simulink model "eVTOL_System"  (R2024b)
settings: Solver=FixedStepAuto  StartTime=0.0  StopTime=inf  RelTol=1e-3
undefined symbols (not defined in the file): airspeed, Battery, BCE12, BCE_Set_init, BMS_Controller_State, C, Cell10_P, Cell11_P, Cell12_P, Cell13_P, Cell14_P, Cell15_P, Cell16_P, Cell17_P, Cell18_P, Cell19_P, Cell1_N, Cell1_P, Cell20_P, Cell21_P, Cell22_P, Cell23_P, Cell24_P, Cell2_P, Cell3_P, Cell4_P, Cell5_P, Cell6_P, Cell7_P, Cell8_P, Cell9_P, Charging_State, CityMission, control, controlParams, ControlSampleTime, CriticalTiltAngle, currentFactor, CV_Gain, ddx, ddy, ddz, Device_01, Device_02, DiscIntNeverNeededParam, dx, dy, dz, Earth, env, F, F28379D_ADC_MaxCount, F28379D_ADC_Vmax, FixedWingMission, flightState, Foc_Ki_IxTcpu, Foc_Ki_S, Foc_Kp_I, Foc_Kp_S, fractalcoef ... (+68)
libraries: fl_lib x1115, nesl_utility x617, slrealtimeethercatlib x217, simulink x130, canmsglib x101, speedgoatlib_IO611_obsolete x91, slpidlib x49, mcbcontrolslib x44, slrealtimeutilitieslib x35, speedgoatlib_hdlCoder_IO3xx x31, dspstat3 x24, mcbpositiondecoderlib x12
(part 21 of 31)

== system eVTOL_System/Flight Controller/Autopilot/Fixed Wing Controller/Fixed Wing Controller Tuning/Attitude Controller/Pitch Roll Controller ==
  note: Small angle assumption. x axis body rate = rate of roll
  note: Inspired by PX4's fixed wing controller
      | https://docs.px4.io/master/en/flight_stack/controller_diagrams.html
  Pitch SP : Inport
  Roll SP : Inport  Port=2
  YPR : Inport  Port=3
  Ang Rate : Inport  Port=4
  Airspeed : Inport  Port=5
  Enable : EnablePort
  Demux : Demux  Outputs=3
  Demux1 : Demux  Outputs=3
  Mux : Mux  Inputs=3
  Pitch Angle Controller : slpidlib/PID Controller  Controller=PID  Form=Parallel  TimeDomain=Discrete-time  UseExternalTs=off  SampleTime=0.005  IntegratorMethod=Forward Euler  FilterMethod=Forward Euler  ControllerParametersSource=internal  P=17.6399272009125  I=10.1914925604101  UseKiTs=off  D=1.4272793655692  UseExternalDerivativeSource=off  N=0.16530941788163  UseFilter=on  TunerSelectOption=Transfer Function Based (PID Tuner App)  InitialConditionSource=internal  InitialConditionForIntegrator=0  InitialConditionForFilter=0  DifferentiatorICPrevScaledInput=0  ExternalReset=none  TrackingMode=off  Kt=1  LimitOutput=on  SatLimitsSource=internal  UpperSaturationLimit=inf  LowerSaturationLimit=-inf  LinearizeAsGain=on  AntiWindupMode=clamping  Kb=1  LimitIntegrator=off  UpperIntegratorSaturationLimit=inf  LowerIntegratorSaturationLimit=-inf  POutMin=[]  POutMax=[]  IOutMin=[]  IOutMax=[]  DOutMin=[]  DOutMax=[]  NOutMin=[]  NOutMax=[]  SumOutMin=[]  SumOutMax=[]  SaturationOutMin=[]  SaturationOutMax=[]  PParamMin=[]  PParamMax=[]  IParamMin=[]  IParamMax=[]  DParamMin=[]  DParamMax=[]  NParamMin=[]  NParamMax=[]  KbParamMin=[]  KbParamMax=[]  KtParamMin=[]  KtParamMax=[]  KbOutMin=[]  KbOutMax=[]  KtOutMin=[]  KtOutMax=[]  IntegratorOutMin=[]  IntegratorOutMax=[]  FilterOutMin=[]  FilterOutMax=[]  SumI1OutMin=[]  SumI1OutMax=[]  SumI2OutMin=[]  SumI2OutMax=[]  SumI3OutMin=[]  SumI3OutMax=[]  SumI4OutMin=[]  SumI4OutMax=[]  SumDOutMin=[]  SumDOutMax=[]  DifferentiatorOutMin=[]  DifferentiatorOutMax=[]  FilterDiffOutCoefMin=[]  FilterDiffOutCoefMax=[]  ReciprocalOutMin=[]  ReciprocalOutMax=[]  SumDenOutMin=[]  SumDenOutMax=[]  SumNumOutMin=[]  SumNumOutMax=[]  DivideOutMin=[]  DivideOutMax=[]  UdiffTsProdOutMin=[]  UdiffTsProdOutMax=[]  NTsProdOutMin=[]  NTsProdOutMax=[]  UintegralTsProdOutMin=[]  UintegralTsProdOutMax=[]  UngainTsProdOutMin=[]  UngainTsProdOutMax=[]  ClampingZeroOutDataTypeStr=Inherit: Inherit via back propagation  ClampingZeroOutMin=[]  ClampingZeroOutMax=[]  FilterDenConstantOutDataTypeStr=Inherit: Inherit via back propagation  FilterDenConstantOutMin=[]  FilterDenConstantOutMax=[]  PCopyOutDataTypeStr=Inherit: Inherit via back propagation  PCopyOutMin=[]  PCopyOutMax=[]  NCopyOutDataTypeStr=Inherit: Inherit via back propagation  NCopyOutMin=[]  NCopyOutMax=[]  IntegratorContinuousStateAttributes=''  IntegratorStateMustResolveToSignalObject=off  IntegratorRTWStateStorageClass=Auto  FilterContinuousStateAttributes=''  FilterStateMustResolveToSignalObject=off  FilterRTWStateStorageClass=Auto  ParallelPVariant=InternalParameters  IdealPVariant=Disabled  IVariant=InternalParameters  DVariant=InternalParameters  IntegratorVariant=Discrete  SatVariant=Enabled  AWVariant=DiscClampingParallel  PCopyVariant=Disabled  TRVariant=Disabled  FdbkBlocksVariant=Forward  IdealPFdbkVariant=Disabled  SatFdbkVariant=Disabled  DerivativeFilterVariant=ForwardEulerFilter  NVariant=InternalParameters  NCopyVariant=Disabled  FilterICVariant=InternalICsFilter  IntegratorICVariant=InternalICs  ExternalResetVariant=Disabled  TRSumVariant=Passthrough  SumFdbkVariant=Disabled  SumVariant=Sum_PID  TsampFilterVariant=InternalTs  TsampNgainVariant=Passthrough  TsampIntegralVariant=Disabled_SignalSpec  ExternalSaturationOutDataTypeStr=Inherit: Same as second input  DerivativeSourceVariant=ErrorSignal  PreIntVariant=InternalPreInt
  Pitch Rate Controller : slpidlib/PID Controller  Controller=P  Form=Parallel  TimeDomain=Discrete-time  UseExternalTs=off  SampleTime=0.005  IntegratorMethod=Forward Euler  FilterMethod=Forward Euler  ControllerParametersSource=internal  P=0.198532533167891  I=0  UseKiTs=off  D=0  UseExternalDerivativeSource=off  N=100  UseFilter=on  TunerSelectOption=Transfer Function Based (PID Tuner App)  InitialConditionSource=internal  InitialConditionForIntegrator=0  InitialConditionForFilter=0  DifferentiatorICPrevScaledInput=0  ExternalReset=either  TrackingMode=off  Kt=1  LimitOutput=on  SatLimitsSource=internal  UpperSaturationLimit=inf  LowerSaturationLimit=-inf  LinearizeAsGain=on  AntiWindupMode=clamping  Kb=1  LimitIntegrator=off  UpperIntegratorSaturationLimit=inf  LowerIntegratorSaturationLimit=-inf  POutMin=[]  POutMax=[]  IOutMin=[]  IOutMax=[]  DOutMin=[]  DOutMax=[]  NOutMin=[]  NOutMax=[]  SumOutMin=[]  SumOutMax=[]  SaturationOutMin=[]  SaturationOutMax=[]  PParamMin=[]  PParamMax=[]  IParamMin=[]  IParamMax=[]  DParamMin=[]  DParamMax=[]  NParamMin=[]  NParamMax=[]  KbParamMin=[]  KbParamMax=[]  KtParamMin=[]  KtParamMax=[]  KbOutMin=[]  KbOutMax=[]  KtOutMin=[]  KtOutMax=[]  IntegratorOutMin=[]  IntegratorOutMax=[]  FilterOutMin=[]  FilterOutMax=[]  SumI1OutMin=[]  SumI1OutMax=[]  SumI2OutMin=[]  SumI2OutMax=[]  SumI3OutMin=[]  SumI3OutMax=[]  SumI4OutMin=[]  SumI4OutMax=[]  SumDOutMin=[]  SumDOutMax=[]  DifferentiatorOutMin=[]  DifferentiatorOutMax=[]  FilterDiffOutCoefMin=[]  FilterDiffOutCoefMax=[]  ReciprocalOutMin=[]  ReciprocalOutMax=[]  SumDenOutMin=[]  SumDenOutMax=[]  SumNumOutMin=[]  SumNumOutMax=[]  DivideOutMin=[]  DivideOutMax=[]  UdiffTsProdOutMin=[]  UdiffTsProdOutMax=[]  NTsProdOutMin=[]  NTsProdOutMax=[]  UintegralTsProdOutMin=[]  UintegralTsProdOutMax=[]  UngainTsProdOutMin=[]  UngainTsProdOutMax=[]  ClampingZeroOutDataTypeStr=Inherit: Inherit via back propagation  ClampingZeroOutMin=[]  ClampingZeroOutMax=[]  FilterDenConstantOutDataTypeStr=Inherit: Inherit via back propagation  FilterDenConstantOutMin=[]  FilterDenConstantOutMax=[]  PCopyOutDataTypeStr=Inherit: Inherit via back propagation  PCopyOutMin=[]  PCopyOutMax=[]  NCopyOutDataTypeStr=Inherit: Inherit via back propagation  NCopyOutMin=[]  NCopyOutMax=[]  IntegratorContinuousStateAttributes=''  IntegratorStateMustResolveToSignalObject=off  IntegratorRTWStateStorageClass=Auto  FilterContinuousStateAttributes=''  FilterStateMustResolveToSignalObject=off  FilterRTWStateStorageClass=Auto  ParallelPVariant=InternalParameters  IdealPVariant=Disabled  IVariant=Disabled  DVariant=Disabled  IntegratorVariant=Disabled  SatVariant=Enabled  AWVariant=Disabled  PCopyVariant=Disabled  TRVariant=Disabled  FdbkBlocksVariant=Forward  IdealPFdbkVariant=Disabled  SatFdbkVariant=Disabled  DerivativeFilterVariant=Disabled  NVariant=Disabled  NCopyVariant=Disabled_SignalSpec  FilterICVariant=Disabled  IntegratorICVariant=Disabled  ExternalResetVariant=Disabled  TRSumVariant=Passthrough  SumFdbkVariant=Disabled  SumVariant=Passthrough_P  TsampFilterVariant=InternalTs  TsampNgainVariant=Passthrough  TsampIntegralVariant=Disabled_SignalSpec  ExternalSaturationOutDataTypeStr=Inherit: Same as second input  DerivativeSourceVariant=Disabled  PreIntVariant=InternalPreInt
  Roll Angle Controller : slpidlib/PID Controller  Controller=P  Form=Parallel  TimeDomain=Discrete-time  UseExternalTs=off  SampleTime=0.005  IntegratorMethod=Forward Euler  FilterMethod=Forward Euler  ControllerParametersSource=internal  P=10.1019363886622  I=0.5  UseKiTs=off  D=2  UseExternalDerivativeSource=off  N=100  UseFilter=on  TunerSelectOption=Transfer Function Based (PID Tuner App)  InitialConditionSource=internal  InitialConditionForIntegrator=0  InitialConditionForFilter=0  DifferentiatorICPrevScaledInput=0  ExternalReset=none  TrackingMode=off  Kt=1  LimitOutput=on  SatLimitsSource=internal  UpperSaturationLimit=control.maxRollRate  LowerSaturationLimit=control.minRollRate  LinearizeAsGain=on  AntiWindupMode=clamping  Kb=1  LimitIntegrator=off  UpperIntegratorSaturationLimit=inf  LowerIntegratorSaturationLimit=-inf  POutMin=[]  POutMax=[]  IOutMin=[]  IOutMax=[]  DOutMin=[]  DOutMax=[]  NOutMin=[]  NOutMax=[]  SumOutMin=[]  SumOutMax=[]  SaturationOutMin=[]  SaturationOutMax=[]  PParamMin=[]  PParamMax=[]  IParamMin=[]  IParamMax=[]  DParamMin=[]  DParamMax=[]  NParamMin=[]  NParamMax=[]  KbParamMin=[]  KbParamMax=[]  KtParamMin=[]  KtParamMax=[]  KbOutMin=[]  KbOutMax=[]  KtOutMin=[]  KtOutMax=[]  IntegratorOutMin=[]  IntegratorOutMax=[]  FilterOutMin=[]  FilterOutMax=[]  SumI1OutMin=[]  SumI1OutMax=[]  SumI2OutMin=[]  SumI2OutMax=[]  SumI3OutMin=[]  SumI3OutMax=[]  SumI4OutMin=[]  SumI4OutMax=[]  SumDOutMin=[]  SumDOutMax=[]  DifferentiatorOutMin=[]  DifferentiatorOutMax=[]  FilterDiffOutCoefMin=[]  FilterDiffOutCoefMax=[]  ReciprocalOutMin=[]  ReciprocalOutMax=[]  SumDenOutMin=[]  SumDenOutMax=[]  SumNumOutMin=[]  SumNumOutMax=[]  DivideOutMin=[]  DivideOutMax=[]  UdiffTsProdOutMin=[]  UdiffTsProdOutMax=[]  NTsProdOutMin=[]  NTsProdOutMax=[]  UintegralTsProdOutMin=[]  UintegralTsProdOutMax=[]  UngainTsProdOutMin=[]  UngainTsProdOutMax=[]  ClampingZeroOutDataTypeStr=Inherit: Inherit via back propagation  ClampingZeroOutMin=[]  ClampingZeroOutMax=[]  FilterDenConstantOutDataTypeStr=Inherit: Inherit via back propagation  FilterDenConstantOutMin=[]  FilterDenConstantOutMax=[]  PCopyOutDataTypeStr=Inherit: Inherit via back propagation  PCopyOutMin=[]  PCopyOutMax=[]  NCopyOutDataTypeStr=Inherit: Inherit via back propagation  NCopyOutMin=[]  NCopyOutMax=[]  IntegratorContinuousStateAttributes=''  IntegratorStateMustResolveToSignalObject=off  IntegratorRTWStateStorageClass=Auto  FilterContinuousStateAttributes=''  FilterStateMustResolveToSignalObject=off  FilterRTWStateStorageClass=Auto  ParallelPVariant=InternalParameters  IdealPVariant=Disabled  IVariant=Disabled  DVariant=Disabled  IntegratorVariant=Disabled  SatVariant=Enabled  AWVariant=Disabled  PCopyVariant=Disabled  TRVariant=Disabled  FdbkBlocksVariant=Forward  IdealPFdbkVariant=Disabled  SatFdbkVariant=Disabled  DerivativeFilterVariant=Disabled  NVariant=Disabled  NCopyVariant=Disabled_SignalSpec  FilterICVariant=Disabled  IntegratorICVariant=Disabled  ExternalResetVariant=Disabled  TRSumVariant=Passthrough  SumFdbkVariant=Disabled  SumVariant=Passthrough_P  TsampFilterVariant=InternalTs  TsampNgainVariant=Passthrough  TsampIntegralVariant=Disabled_SignalSpec  ExternalSaturationOutDataTypeStr=Inherit: Same as second input  DerivativeSourceVariant=Disabled  PreIntVariant=InternalPreInt
  Roll Rate Controller : slpidlib/PID Controller  Controller=PI  Form=Parallel  TimeDomain=Discrete-time  UseExternalTs=off  SampleTime=0.005  IntegratorMethod=Forward Euler  FilterMethod=Forward Euler  ControllerParametersSource=internal  P=0.1457375768301  I=3.00000582031009  UseKiTs=off  D=2  UseExternalDerivativeSource=off  N=100  UseFilter=on  TunerSelectOption=Transfer Function Based (PID Tuner App)  InitialConditionSource=internal  InitialConditionForIntegrator=0  InitialConditionForFilter=0  DifferentiatorICPrevScaledInput=0  ExternalReset=none  TrackingMode=off  Kt=1  LimitOutput=on  SatLimitsSource=internal  UpperSaturationLimit=1  LowerSaturationLimit=-1  LinearizeAsGain=on  AntiWindupMode=clamping  Kb=1  LimitIntegrator=off  UpperIntegratorSaturationLimit=inf  LowerIntegratorSaturationLimit=-inf  POutMin=[]  POutMax=[]  IOutMin=[]  IOutMax=[]  DOutMin=[]  DOutMax=[]  NOutMin=[]  NOutMax=[]  SumOutMin=[]  SumOutMax=[]  SaturationOutMin=[]  SaturationOutMax=[]  PParamMin=[]  PParamMax=[]  IParamMin=[]  IParamMax=[]  DParamMin=[]  DParamMax=[]  NParamMin=[]  NParamMax=[]  KbParamMin=[]  KbParamMax=[]  KtParamMin=[]  KtParamMax=[]  KbOutMin=[]  KbOutMax=[]  KtOutMin=[]  KtOutMax=[]  IntegratorOutMin=[]  IntegratorOutMax=[]  FilterOutMin=[]  FilterOutMax=[]  SumI1OutMin=[]  SumI1OutMax=[]  SumI2OutMin=[]  SumI2OutMax=[]  SumI3OutMin=[]  SumI3OutMax=[]  SumI4OutMin=[]  SumI4OutMax=[]  SumDOutMin=[]  SumDOutMax=[]  DifferentiatorOutMin=[]  DifferentiatorOutMax=[]  FilterDiffOutCoefMin=[]  FilterDiffOutCoefMax=[]  ReciprocalOutMin=[]  ReciprocalOutMax=[]  SumDenOutMin=[]  SumDenOutMax=[]  SumNumOutMin=[]  SumNumOutMax=[]  DivideOutMin=[]  DivideOutMax=[]  UdiffTsProdOutMin=[]  UdiffTsProdOutMax=[]  NTsProdOutMin=[]  NTsProdOutMax=[]  UintegralTsProdOutMin=[]  UintegralTsProdOutMax=[]  UngainTsProdOutMin=[]  UngainTsProdOutMax=[]  ClampingZeroOutDataTypeStr=Inherit: Inherit via back propagation  ClampingZeroOutMin=[]  ClampingZeroOutMax=[]  FilterDenConstantOutDataTypeStr=Inherit: Inherit via back propagation  FilterDenConstantOutMin=[]  FilterDenConstantOutMax=[]  PCopyOutDataTypeStr=Inherit: Inherit via back propagation  PCopyOutMin=[]  PCopyOutMax=[]  NCopyOutDataTypeStr=Inherit: Inherit via back propagation  NCopyOutMin=[]  NCopyOutMax=[]  IntegratorContinuousStateAttributes=''  IntegratorStateMustResolveToSignalObject=off  IntegratorRTWStateStorageClass=Auto  FilterContinuousStateAttributes=''  FilterStateMustResolveToSignalObject=off  FilterRTWStateStorageClass=Auto  ParallelPVariant=InternalParameters  IdealPVariant=Disabled  IVariant=InternalParameters  DVariant=Disabled  IntegratorVariant=Discrete  SatVariant=Enabled  AWVariant=DiscClampingParallel  PCopyVariant=Disabled  TRVariant=Disabled  FdbkBlocksVariant=Forward  IdealPFdbkVariant=Disabled  SatFdbkVariant=Disabled  DerivativeFilterVariant=Disabled  NVariant=Disabled  NCopyVariant=Disabled_SignalSpec  FilterICVariant=Disabled  IntegratorICVariant=InternalICs  ExternalResetVariant=Disabled  TRSumVariant=Passthrough  SumFdbkVariant=Disabled  SumVariant=Sum_PI  TsampFilterVariant=InternalTs  TsampNgainVariant=Passthrough  TsampIntegralVariant=Disabled_SignalSpec  ExternalSaturationOutDataTypeStr=Inherit: Same as second input  DerivativeSourceVariant=Disabled  PreIntVariant=InternalPreInt
  Saturation : Saturate  UpperLimit=control.maxRoll  LowerLimit=control.minRoll
  Saturation1 : Saturate  UpperLimit=control.maxPitch  LowerLimit=control.minPitch
  Saturation2 : Saturate  UpperLimit=0.3  LowerLimit=-0.3
  Sum{,1..3} (4 alike) : Sum  Inputs=|+-
  Terminator : Terminator
  Turn Coordinator : Subsystem
  Unary Minus1 : UnaryMinus
  AER : Outport
  wires:
  Sum/1 -> Pitch Angle Controller/1
  YPR/1 -> Demux/1
  Demux/2 -> Sum/2
  Mux/1 -> AER/1
  Saturation1/1 -> Sum/1, Turn Coordinator/2(Pitch SP)
  Ang Rate/1 -> Demux1/1
  Pitch SP/1 -> Saturation1/1
  Pitch Rate Controller/1 -> Unary Minus1/1
  Demux/3 -> Sum1/2
  Saturation/1 -> Sum1/1, Turn Coordinator/1(Roll SP)
  Roll SP/1 -> Saturation/1
  Sum1/1 -> Roll Angle Controller/1
  Demux/1 -> Terminator/1
  Airspeed/1 -> Turn Coordinator/3(Airspeed)
  Demux1/3 -> Turn Coordinator/4(r)
  Turn Coordinator/1(Rudder) -> Mux/3  "dR"
  Unary Minus1/1 -> Mux/2  "dE"
  Saturation2/1 -> Mux/1
  Sum2/1 -> Roll Rate Controller/1
  Roll Angle Controller/1 -> Sum2/1
  Demux1/1 -> Sum2/2
  Roll Rate Controller/1 -> Saturation2/1
  Demux1/2 -> Sum3/2
  Pitch Angle Controller/1 -> Sum3/1
  Sum3/1 -> Pitch Rate Controller/1

== system eVTOL_System/Flight Controller/Autopilot/Fixed Wing Controller/Fixed Wing Controller Tuning/Attitude Controller/Rudder Heading Controller ==
  note: Rudder control during takeoff ground-run.
      | Not implemented currently.
  Yaw SP : Inport
  YPR : Inport  Port=2
  Ang Rate : Inport  Port=3
  Enable : EnablePort
  Constant : Constant  Value=0
  Constant1 : Constant  Value=0
  Mux : Mux  Inputs=3
  Selector : Selector  InputPortWidth=3  IndexOptions=Index vector (dialog)  Indices=1  OutputSizes=1
  Selector1 : Selector  InputPortWidth=3  IndexOptions=Index vector (dialog)  Indices=3  OutputSizes=1
  Terminator : Terminator
  Terminator1 : Terminator
  Terminator2 : Terminator
  AER : Outport
  wires:
  YPR/1 -> Selector/1
  Mux/1 -> AER/1
  Constant/1 -> Mux/2, Mux/1
  Ang Rate/1 -> Selector1/1
  Constant1/1 -> Mux/3
  Yaw SP/1 -> Terminator/1
  Selector/1 -> Terminator1/1
  Selector1/1 -> Terminator2/1

== system eVTOL_System/Flight Controller/Autopilot/Multicopter Controller/Attitude Control/Derivative Gain/Pitch Ref Deriv ==
  In1 : Inport
  Discrete-Time Integrator : DiscreteIntegrator  SampleTime=-1  ICPrevOutput=DiscIntNeverNeededParam  ICPrevScaledInput=DiscIntNeverNeededParam
  Gain : Gain  Gain=controlParams.N_PITCH
  Sum : Sum  Inputs=|+-
  Out1 : Outport
  wires:
  Gain/1 -> Out1/1, Discrete-Time Integrator/1
  In1/1 -> Sum/1
  Sum/1 -> Gain/1
  Discrete-Time Integrator/1 -> Sum/2

== system eVTOL_System/Flight Controller/Autopilot/Multicopter Controller/Attitude Control/Derivative Gain/Roll Ref Deriv ==
  In1 : Inport
  Discrete-Time Integrator : DiscreteIntegrator  SampleTime=-1  ICPrevOutput=DiscIntNeverNeededParam  ICPrevScaledInput=DiscIntNeverNeededParam
  Gain : Gain  Gain=controlParams.N_ROLL
  Sum : Sum  Inputs=|+-
  Out1 : Outport
  wires:
  Discrete-Time Integrator/1 -> Sum/2
  Sum/1 -> Gain/1
  In1/1 -> Sum/1
  Gain/1 -> Discrete-Time Integrator/1, Out1/1

== system eVTOL_System/Flight Controller/Guidance Test Bench/ControlType/Guidance Testbench/Guidance Logic/Guidance Stateflow ==
  note: Can be replaced with a signal from the GCS to "Start Mission"
  Pose : Inport
  GCSCommands : Inport  Port=2
  LandingStates : Inport  Port=3
  States : Inport  Port=4
  "Bus " : BusSelector  OutputSignals=LAP,YawCmd
  Bus Selector : BusSelector  OutputSignals=mode
  Compare To Constant : simulink/Logic and Bit Operations/Compare To Constant  relop===  const=1  OutDataTypeStr=boolean
  Constant : Constant  Value=FSState
  Delay : Delay  DelayLength=1  InitialCondition=0
  Guidance Mode Selector : Stateflow chart  TreatAsAtomicUnit=on  SystemSampleTime=0.02
      settings: PortSchema="{\"entries\":[{\"content\":{\"sides\":[{\"content\":{\"connectorIds\":[\"In1\",\"In2\",\"In3\",\"In4\",\"In5\",\"In6\"]},\"type\":\"ConnectorPlacement.EquallySpacedRectSide\",\"uuid\":\"a9cfd0e2-196c-422d-b359-9161a47768c9\"},{\"content\":{\"connectorIds\":[\"Out7\",\"Out2\",\"Out3\",\"Out4\",\"Out5\",\"Out6\",\"Out1\"],\"side\":\"RIGHT\"},\"type\":\"ConnectorPlacement.EquallySpacedRectSide\",\"uuid\":\"4fed41ae-e7cf-4de3-8bdb-9e24e7d8b079\"},{\"content\":{\"side\":\"TOP\"},\"type\":\"ConnectorPlacement.EquallySpacedRectSide\",\"uuid\":\"2d49ff20-2f63-498d-ac9d-820eae01f794\"}]},\"type\":\"ConnectorPlacement.EquallySpacedConnector\",\"uuid\":\"88d403f4-ad96-40f9-9697-84906f26a8bf\"}],\"packageUris\":[\"http://schema.mathworks.com/mf0/Connector/R2020b\"],\"version\":\"1.0\"}"
  Home : Constant  Value=[0 0 0]  OutDataTypeStr=double
  Landed? : simulink/Logic and Bit Operations/Compare To Constant  relop===  const=2  OutDataTypeStr=boolean
  MissionAction : Constant  Value=0  OutDataTypeStr=uint8
  Mux : Mux  Inputs=2
  Rate Transition : RateTransition
  Rate Transition1 : RateTransition
  Rate Transition2 : RateTransition
  "Select \"From\" Waypoint" : Selector  InputPortWidth=2  IndexOptions=Index vector (dialog)  Indices=2  OutputSizes=1
  "Select \"To\" Waypoint" : Selector  InputPortWidth=2  IndexOptions=Index vector (dialog)  Indices=1  OutputSizes=1
  Stop Simulation : Stop
  Takeoff IC : InitialCondition
  Terminator : Terminator
  UAV Path Manager : uavalgslib/Path Manager  UAVType=multirotor  LoiterRadius=25  dataType=double  inputBusName='doubleUavPathManager'  SimulateUsing=Code generation
  HoverCommands : Outport
  AACSP : Outport  Port=2
  FixedWingSP : Outport  Port=3
  ctrlMode : Outport  Port=4
  FlightMode : Outport  Port=5
  wires:
  Takeoff IC/1 -> Guidance Mode Selector/1(mode)
  MissionAction/1 -> UAV Path Manager/4
  Guidance Mode Selector/1(Status) -> Delay/1, Landed?/1
  Home/1 -> UAV Path Manager/5
  GCSCommands/1 -> Rate Transition2/1
  Pose/1 -> Rate Transition1/1
  UAV Path Manager/1 -> Rate Transition/1
  Bus Selector/1 -> Takeoff IC/1  "<mode>"
  [pose] -> Guidance Mode Selector/4(Pose)
  Compare To Constant/1 -> UAV Path Manager/3
  "Select \"To\" Waypoint"/1 -> Guidance Mode Selector/2(ToWP), Bus Selector/1
  "Select \"From\" Waypoint"/1 -> Guidance Mode Selector/3(FromWP)
  Landed?/1 -> Stop Simulation/1
  Guidance Mode Selector/2(GdncMode) -> Terminator/1
  Delay/1 -> Compare To Constant/1
  LandingStates/1 -> [landingState]
  States/1 -> Guidance Mode Selector/5(States)
  Guidance Mode Selector/5(controlMode) -> ctrlMode/1
  Guidance Mode Selector/3(aacSP) -> AACSP/1
  Guidance Mode Selector/4(FixedWingSP) -> FixedWingSP/1
  Guidance Mode Selector/6(FlightMode) -> FlightMode/1
  Constant/1 -> Guidance Mode Selector/6(PresetMode)
  "Bus "/1 -> Mux/1  "<LAP>"
  "Bus "/2 -> Mux/2  "<YawCmd>"
  Mux/1 -> HoverCommands/1
  Guidance Mode Selector/7(InnerLoopCmds) -> "Bus "/1
  Rate Transition/1 -> "Select \"From\" Waypoint"/1, "Select \"To\" Waypoint"/1
  Rate Transition1/1 -> UAV Path Manager/1, [pose]
  Rate Transition2/1 -> UAV Path Manager/2

== system eVTOL_System/Flight Controller/Guidance Test Bench/ControlType/Guidance Testbench/Guidance Logic/Interface ==
  UAVState : Inport
  Bus Creator : BusCreator  Inputs=5
  Bus Selector : BusSelector  OutputSignals=Xe,Ve
  Demux : Demux  Outputs=3
  Selector : Selector  InputPortWidth=3  IndexOptions=Index vector (dialog)  Indices=[1]  OutputSizes=1
  Selector1 : Selector  InputPortWidth=3  IndexOptions=Index vector (dialog)  Indices=[2]  OutputSizes=1
  States : Outport
  wires:
  Demux/2 -> Bus Creator/2  "y"
  UAVState/1 -> Bus Selector/1
  Bus Selector/2 -> Selector/1, Selector1/1  "<Ve>"
  Bus Selector/1 -> Demux/1  "<Xe>"
  Demux/1 -> Bus Creator/1  "x"
  Selector/1 -> Bus Creator/4  "vx"
  Demux/3 -> Bus Creator/3  "z"
  Selector1/1 -> Bus Creator/5  "vy"
  Bus Creator/1 -> States/1

== system eVTOL_System/Flight Controller/Guidance Test Bench/ControlType/Guidance Testbench/Guidance Logic/Subsystem ==
  note: Tilt Angle also determines the state aircraft is in. Thus a unit delay is added
  UAVState : Inport
  Bus Creator : BusCreator  Inputs=6  OutDataTypeStr=Bus: GuidanceStates
  Bus Selector : BusSelector  OutputSignals=Euler,pqr,Ve,Xe,course,RotorParameters.Rotor A
  Gain : Gain
  Unit Delay : UnitDelay  InitialCondition=tiltIni  SampleTime=-1  HasFrameUpgradeWarning=on
  States : Outport
  wires:
  UAVState/1 -> Bus Selector/1
  Bus Selector/1 -> Bus Creator/1  "<Euler>"
  Bus Creator/1 -> States/1
  Bus Selector/3 -> Bus Creator/3  "<Ve>"
  Bus Selector/2 -> Bus Creator/2  "<pqr>"
  Bus Selector/4 -> Bus Creator/4  "<Xe>"
  Bus Selector/5 -> Bus Creator/5  "<course>"
  Bus Selector/6 -> Unit Delay/1  "<Rotor A>"
  Gain/1 -> Bus Creator/6  "Tilt"
  Unit Delay/1 -> Gain/1  "Tilt2"

== system eVTOL_System/Flight Controller/Guidance Test Bench/ControlType/Manual Control/Command Interface/Control Rate Transition ==
  FM : Inport
  "ControlMode " : Inport  Port=2
  FixedWingSetpoint : Inport  Port=3
  AACSetpoint : Inport  Port=4
  Position : Inport  Port=5
  Rate Transition{,1..3,5} (5 alike) : RateTransition  OutPortSampleTime=ControlSampleTime
  ctrlMode : Outport
  FixedWingSP : Outport  Port=2
  AACSP : Outport  Port=3
  PositionCmds : Outport  Port=4
  FlightMode : Outport  Port=5
  wires:
  Rate Transition5/1 -> FlightMode/1
  Position/1 -> Rate Transition3/1
  FixedWingSetpoint/1 -> Rate Transition1/1
  Rate Transition3/1 -> PositionCmds/1
  FM/1 -> Rate Transition5/1
  "ControlMode "/1 -> Rate Transition/1
  Rate Transition1/1 -> FixedWingSP/1
  AACSetpoint/1 -> Rate Transition2/1
  Rate Transition2/1 -> AACSP/1
  Rate Transition/1 -> ctrlMode/1

== system eVTOL_System/Flight Controller/Guidance Test Bench/ControlType/Manual Control/Command Interface/Subsystem ==
  note: Tilt Angle also determines the state aircraft is in. Thus a unit delay is added
  UAVState : Inport
  Bus Creator : BusCreator  Inputs=6  OutDataTypeStr=Bus: GuidanceStates
  Bus Selector : BusSelector  OutputSignals=Euler,pqr,Ve,Xe,course,RotorParameters.Rotor A
  Gain : Gain
  Unit Delay : UnitDelay  InitialCondition=tiltIni  SampleTime=-1  HasFrameUpgradeWarning=on
  States : Outport
  wires:
  UAVState/1 -> Bus Selector/1
  Bus Selector/1 -> Bus Creator/1  "<Euler>"
  Bus Creator/1 -> States/1
  Bus Selector/3 -> Bus Creator/3  "<Ve>"
  Bus Selector/2 -> Bus Creator/2  "<pqr>"
  Bus Selector/4 -> Bus Creator/4  "<Xe>"
  Bus Selector/5 -> Bus Creator/5  "<course>"
  Bus Selector/6 -> Unit Delay/1  "<Rotor A>"
  Gain/1 -> Bus Creator/6  "Tilt"
  Unit Delay/1 -> Gain/1  "Tilt2"

== system eVTOL_System/Motor Drive/Controller/Controller_MIL/F28379D Firmware/Controller Algorithm/FOC ==
  note: Field-Oriented Control for PMSM
  Iab : Inport
  Pos : Inport  Port=2
  Speedfb : Inport  Port=3
  EnClosedLoop : Inport  Port=4
  SpeedRef : Inport  Port=5
  EnablePWM : Inport  Port=6
  Kp_S : Inport  Port=7
  Ki_S : Inport  Port=8
  Kp_i : Inport  Port=9
  Ki_ixTcpu : Inport  Port=10
  Current Control : Subsystem  TreatAsAtomicUnit=on
  Data Type Conversion : DataTypeConversion  OutDataTypeStr=boolean  SaturateOnIntegerOverflow=off  RndMeth=Floor
  Mux : Mux  Inputs=2
  RT{1,3..5} (4 alike) : RateTransition  Deterministic=off  OutPortSampleTime=Ts_speed
  RT2 : RateTransition  Deterministic=off
  RT6 : RateTransition  Deterministic=off
  RT7 : RateTransition  Deterministic=off
  Speed Control MLD : Subsystem
  ModWave : Outport
  PWM_Enable : Outport  Port=2
  wires:
  Speed Control MLD/1(IdqRef_PU) -> RT2/1
  EnClosedLoop/1 -> Mux/1, RT5/1
  Speedfb/1 -> RT1/1
  Current Control/2(PWM_Enable) -> Data Type Conversion/1
  EnablePWM/1 -> Mux/2, RT4/1
  Ki_S/1 -> Speed Control MLD/6(Ki_S)
  Current Control/1(ModWave) -> ModWave/1
  Iab/1 -> Current Control/1(Iab)
  Kp_S/1 -> Speed Control MLD/5(Kp_S)
  Pos/1 -> Current Control/2(Pos)
  SpeedRef/1 -> RT6/1, RT3/1
  Mux/1 -> RT7/1
  RT2/1 -> Current Control/4(Idq_ref_PU)
  RT6/1 -> Current Control/5(SpeedRef)
  RT7/1 -> Current Control/3(Enable)
  RT1/1 -> Speed Control MLD/4(Speed_Meas_PU)
  RT3/1 -> Speed Control MLD/3(SpeedRef)
  Data Type Conversion/1 -> PWM_Enable/1
  RT5/1 -> Speed Control MLD/1(En_closedloop)
  RT4/1 -> Speed Control MLD/2(EnablePWM)
  Kp_i/1 -> Current Control/6(Kp_i)
  Ki_ixTcpu/1 -> Current Control/7(Ki_ixTcpu)

== system eVTOL_System/Motor Drive/Controller/Controller_MIL/F28379D Firmware/Controller Algorithm/Speed and Pos Decoder ==
  QEP_Position_Count : Inport
  QEP_Index_Latch : Inport  Port=2
  Offset : Inport  Port=3
  Delay : Delay  DelayLength=1
  IIR Filter : mcbcontrolslib/IIR Filter  VariantControl=Low Pass Filter  VariantSelect=Low-pass  FilterConstantInputType=Specify via dialog  Filter_constant=0.01  advancedSettings=off  Ts=50e-6  cutOff_freq=32.1525
  IndexFinder : Subsystem
  Mechanical to Electrical Position : mcbpositiondecoderlib/Mechanical to Electrical Position  PolePairsInputType=Specify via dialog  NrPP=Maxon_645604_Np  selectedRange=Per unit  MechOfstInputType=Input port  mechOffsetIn=0  maxAngleIn=1  InputDataType=single  VariantSelect=floating-point
  NOT : Logic  Operator=NOT  AllPortsSameDT=off  OutDataTypeStr=boolean
  Quadrature Decoder : mcbpositiondecoderlib/Quadrature Decoder  EncoderSlitsPerRevolution=Maxon_Mile_Nslits  EncoderCountsPerSlit=4  CounterSize=16 bits  ExternalIndexCount=on  PositionUnit=Per unit  PositionDataType=single  ParameterInputType=off  CountsPerRevInverseDataType=single
  Speed Measurement : mcbpositiondecoderlib/Speed Measurement  PositionUnit=Per unit  PositionScalingDatatype=uint32  SpeedCalculationMode=Time interval for speed calculation  SampleTimeAsync=Ts_CPU  MaximumApplicationSpeed=6000  SpeedResolution=5e-6  DelayLength=20  MaximumMeasurableSpeed=29999  MeasurableSpeedResolution=1.397e-05  SpeedUnit=Per unit based on dialog  PerUnitSpeed=PU_System_N_base  SpeedDataType=single
  Theta_e : Outport  VectorParamsAs1DForOutWhenUnconnected=off
  speed : Outport  Port=2  VectorParamsAs1DForOutWhenUnconnected=off
  IndexFound : Outport  Port=3  InitialOutput=0  VectorParamsAs1DForOutWhenUnconnected=off
  wires:
  Mechanical to Electrical Position/1 -> Theta_e/1  "Pos"
  Speed Measurement/1 -> IIR Filter/1
  Quadrature Decoder/1 -> Speed Measurement/1, Mechanical to Electrical Position/1
  QEP_Position_Count/1 -> Quadrature Decoder/1
  Offset/1 -> Mechanical to Electrical Position/2
  IIR Filter/1 -> speed/1
  NOT/1 -> IndexFinder/Enable
  QEP_Index_Latch/1 -> IndexFinder/1(In1), Quadrature Decoder/2
  Delay/1 -> NOT/1
  IndexFinder/1(IndexFound) -> IndexFound/1, Delay/1

== system eVTOL_System/Motor Drive/Controller1/Controller_MIL/F28379D Firmware/Controller Algorithm/FOC ==
  note: Field-Oriented Control for PMSM
  Iab : Inport
  Pos : Inport  Port=2
  Speedfb : Inport  Port=3
  EnClosedLoop : Inport  Port=4
  SpeedRef : Inport  Port=5
  EnablePWM : Inport  Port=6
  Kp_S : Inport  Port=7
  Ki_S : Inport  Port=8
  Kp_i : Inport  Port=9
  Ki_ixTcpu : Inport  Port=10
  Current Control : Subsystem  TreatAsAtomicUnit=on
  Data Type Conversion : DataTypeConversion  OutDataTypeStr=boolean  SaturateOnIntegerOverflow=off  RndMeth=Floor
  Mux : Mux  Inputs=2
  RT{1,3..5} (4 alike) : RateTransition  Deterministic=off  OutPortSampleTime=Ts_speed
  RT2 : RateTransition  Deterministic=off
  RT6 : RateTransition  Deterministic=off
  RT7 : RateTransition  Deterministic=off
  Speed Control MLD : Subsystem
  ModWave : Outport
  PWM_Enable : Outport  Port=2
  wires:
  Speed Control MLD/1(IdqRef_PU) -> RT2/1
  EnClosedLoop/1 -> Mux/1, RT5/1
  Speedfb/1 -> RT1/1
  Current Control/2(PWM_Enable) -> Data Type Conversion/1
  EnablePWM/1 -> Mux/2, RT4/1
  Ki_S/1 -> Speed Control MLD/6(Ki_S)
  Current Control/1(ModWave) -> ModWave/1
  Iab/1 -> Current Control/1(Iab)
  Kp_S/1 -> Speed Control MLD/5(Kp_S)
  Pos/1 -> Current Control/2(Pos)
  SpeedRef/1 -> RT6/1, RT3/1
  Mux/1 -> RT7/1
  RT2/1 -> Current Control/4(Idq_ref_PU)
  RT6/1 -> Current Control/5(SpeedRef)
  RT7/1 -> Current Control/3(Enable)
  RT1/1 -> Speed Control MLD/4(Speed_Meas_PU)
  RT3/1 -> Speed Control MLD/3(SpeedRef)
  Data Type Conversion/1 -> PWM_Enable/1
  RT5/1 -> Speed Control MLD/1(En_closedloop)
  RT4/1 -> Speed Control MLD/2(EnablePWM)
  Kp_i/1 -> Current Control/6(Kp_i)
  Ki_ixTcpu/1 -> Current Control/7(Ki_ixTcpu)

== system eVTOL_System/Motor Drive/Controller1/Controller_MIL/F28379D Firmware/Controller Algorithm/Speed and Pos Decoder ==
  QEP_Position_Count : Inport
  QEP_Index_Latch : Inport  Port=2
  Offset : Inport  Port=3
  Delay : Delay  DelayLength=1
  IIR Filter : mcbcontrolslib/IIR Filter  VariantControl=Low Pass Filter  VariantSelect=Low-pass  FilterConstantInputType=Specify via dialog  Filter_constant=0.01  advancedSettings=off  Ts=50e-6  cutOff_freq=32.1525
  IndexFinder : Subsystem
  Mechanical to Electrical Position : mcbpositiondecoderlib/Mechanical to Electrical Position  PolePairsInputType=Specify via dialog  NrPP=Maxon_645604_Np  selectedRange=Per unit  MechOfstInputType=Input port  mechOffsetIn=0  maxAngleIn=1  InputDataType=single  VariantSelect=floating-point
  NOT : Logic  Operator=NOT  AllPortsSameDT=off  OutDataTypeStr=boolean
  Quadrature Decoder : mcbpositiondecoderlib/Quadrature Decoder  EncoderSlitsPerRevolution=Maxon_Mile_Nslits  EncoderCountsPerSlit=4  CounterSize=16 bits  ExternalIndexCount=on  PositionUnit=Per unit  PositionDataType=single  ParameterInputType=off  CountsPerRevInverseDataType=single
  Speed Measurement : mcbpositiondecoderlib/Speed Measurement  PositionUnit=Per unit  PositionScalingDatatype=uint32  SpeedCalculationMode=Time interval for speed calculation  SampleTimeAsync=Ts_CPU  MaximumApplicationSpeed=6000  SpeedResolution=5e-6  DelayLength=20  MaximumMeasurableSpeed=29999  MeasurableSpeedResolution=1.397e-05  SpeedUnit=Per unit based on dialog  PerUnitSpeed=PU_System_N_base  SpeedDataType=single
  Theta_e : Outport  VectorParamsAs1DForOutWhenUnconnected=off
  speed : Outport  Port=2  VectorParamsAs1DForOutWhenUnconnected=off
  IndexFound : Outport  Port=3  InitialOutput=0  VectorParamsAs1DForOutWhenUnconnected=off
  wires:
  Mechanical to Electrical Position/1 -> Theta_e/1  "Pos"
  Speed Measurement/1 -> IIR Filter/1
  Quadrature Decoder/1 -> Speed Measurement/1, Mechanical to Electrical Position/1
  QEP_Position_Count/1 -> Quadrature Decoder/1
  Offset/1 -> Mechanical to Electrical Position/2
  IIR Filter/1 -> speed/1
  NOT/1 -> IndexFinder/Enable
  QEP_Index_Latch/1 -> IndexFinder/1(In1), Quadrature Decoder/2
  Delay/1 -> NOT/1
  IndexFinder/1(IndexFound) -> IndexFound/1, Delay/1

== system eVTOL_System/Motor Drive/Controller2/Controller_MIL/F28379D Firmware/Controller Algorithm/FOC ==
  note: Field-Oriented Control for PMSM
  Iab : Inport
  Pos : Inport  Port=2
  Speedfb : Inport  Port=3
  EnClosedLoop : Inport  Port=4
  SpeedRef : Inport  Port=5
  EnablePWM : Inport  Port=6
  Kp_S : Inport  Port=7
  Ki_S : Inport  Port=8
  Kp_i : Inport  Port=9
  Ki_ixTcpu : Inport  Port=10
  Current Control : Subsystem  TreatAsAtomicUnit=on
  Data Type Conversion : DataTypeConversion  OutDataTypeStr=boolean  SaturateOnIntegerOverflow=off  RndMeth=Floor
  Mux : Mux  Inputs=2
  RT{1,3..5} (4 alike) : RateTransition  Deterministic=off  OutPortSampleTime=Ts_speed
  RT2 : RateTransition  Deterministic=off
  RT6 : RateTransition  Deterministic=off
  RT7 : RateTransition  Deterministic=off
  Speed Control MLD : Subsystem
  ModWave : Outport
  PWM_Enable : Outport  Port=2
  wires:
  Speed Control MLD/1(IdqRef_PU) -> RT2/1
  EnClosedLoop/1 -> Mux/1, RT5/1
  Speedfb/1 -> RT1/1
  Current Control/2(PWM_Enable) -> Data Type Conversion/1
  EnablePWM/1 -> Mux/2, RT4/1
  Ki_S/1 -> Speed Control MLD/6(Ki_S)
  Current Control/1(ModWave) -> ModWave/1
  Iab/1 -> Current Control/1(Iab)
  Kp_S/1 -> Speed Control MLD/5(Kp_S)
  Pos/1 -> Current Control/2(Pos)
  SpeedRef/1 -> RT6/1, RT3/1
  Mux/1 -> RT7/1
  RT2/1 -> Current Control/4(Idq_ref_PU)
  RT6/1 -> Current Control/5(SpeedRef)
  RT7/1 -> Current Control/3(Enable)
  RT1/1 -> Speed Control MLD/4(Speed_Meas_PU)
  RT3/1 -> Speed Control MLD/3(SpeedRef)
  Data Type Conversion/1 -> PWM_Enable/1
  RT5/1 -> Speed Control MLD/1(En_closedloop)
  RT4/1 -> Speed Control MLD/2(EnablePWM)
  Kp_i/1 -> Current Control/6(Kp_i)
  Ki_ixTcpu/1 -> Current Control/7(Ki_ixTcpu)

== system eVTOL_System/Motor Drive/Controller2/Controller_MIL/F28379D Firmware/Controller Algorithm/Speed and Pos Decoder ==
  QEP_Position_Count : Inport
  QEP_Index_Latch : Inport  Port=2
  Offset : Inport  Port=3
  Delay : Delay  DelayLength=1
  IIR Filter : mcbcontrolslib/IIR Filter  VariantControl=Low Pass Filter  VariantSelect=Low-pass  FilterConstantInputType=Specify via dialog  Filter_constant=0.01  advancedSettings=off  Ts=50e-6  cutOff_freq=32.1525
  IndexFinder : Subsystem
  Mechanical to Electrical Position : mcbpositiondecoderlib/Mechanical to Electrical Position  PolePairsInputType=Specify via dialog  NrPP=Maxon_645604_Np  selectedRange=Per unit  MechOfstInputType=Input port  mechOffsetIn=0  maxAngleIn=1  InputDataType=single  VariantSelect=floating-point
  NOT : Logic  Operator=NOT  AllPortsSameDT=off  OutDataTypeStr=boolean
  Quadrature Decoder : mcbpositiondecoderlib/Quadrature Decoder  EncoderSlitsPerRevolution=Maxon_Mile_Nslits  EncoderCountsPerSlit=4  CounterSize=16 bits  ExternalIndexCount=on  PositionUnit=Per unit  PositionDataType=single  ParameterInputType=off  CountsPerRevInverseDataType=single
  Speed Measurement : mcbpositiondecoderlib/Speed Measurement  PositionUnit=Per unit  PositionScalingDatatype=uint32  SpeedCalculationMode=Time interval for speed calculation  SampleTimeAsync=Ts_CPU  MaximumApplicationSpeed=6000  SpeedResolution=5e-6  DelayLength=20  MaximumMeasurableSpeed=29999  MeasurableSpeedResolution=1.397e-05  SpeedUnit=Per unit based on dialog  PerUnitSpeed=PU_System_N_base  SpeedDataType=single
  Theta_e : Outport  VectorParamsAs1DForOutWhenUnconnected=off
  speed : Outport  Port=2  VectorParamsAs1DForOutWhenUnconnected=off
  IndexFound : Outport  Port=3  InitialOutput=0  VectorParamsAs1DForOutWhenUnconnected=off
  wires:
  Mechanical to Electrical Position/1 -> Theta_e/1  "Pos"
  Speed Measurement/1 -> IIR Filter/1
  Quadrature Decoder/1 -> Speed Measurement/1, Mechanical to Electrical Position/1
  QEP_Position_Count/1 -> Quadrature Decoder/1
  Offset/1 -> Mechanical to Electrical Position/2
  IIR Filter/1 -> speed/1
  NOT/1 -> IndexFinder/Enable
  QEP_Index_Latch/1 -> IndexFinder/1(In1), Quadrature Decoder/2
  Delay/1 -> NOT/1
  IndexFinder/1(IndexFound) -> IndexFound/1, Delay/1

== system eVTOL_System/Motor Drive/Controller3/Controller_MIL/F28379D Firmware/Controller Algorithm/FOC ==
  note: Field-Oriented Control for PMSM
  Iab : Inport
  Pos : Inport  Port=2
  Speedfb : Inport  Port=3
  EnClosedLoop : Inport  Port=4
  SpeedRef : Inport  Port=5
  EnablePWM : Inport  Port=6
  Kp_S : Inport  Port=7
  Ki_S : Inport  Port=8
  Kp_i : Inport  Port=9
  Ki_ixTcpu : Inport  Port=10
  Current Control : Subsystem  TreatAsAtomicUnit=on
  Data Type Conversion : DataTypeConversion  OutDataTypeStr=boolean  SaturateOnIntegerOverflow=off  RndMeth=Floor
  Mux : Mux  Inputs=2
  RT{1,3..5} (4 alike) : RateTransition  Deterministic=off  OutPortSampleTime=Ts_speed
  RT2 : RateTransition  Deterministic=off
  RT6 : RateTransition  Deterministic=off
  RT7 : RateTransition  Deterministic=off
  Speed Control MLD : Subsystem
  ModWave : Outport
  PWM_Enable : Outport  Port=2
  wires:
  Speed Control MLD/1(IdqRef_PU) -> RT2/1
  EnClosedLoop/1 -> Mux/1, RT5/1
  Speedfb/1 -> RT1/1
  Current Control/2(PWM_Enable) -> Data Type Conversion/1
  EnablePWM/1 -> Mux/2, RT4/1
  Ki_S/1 -> Speed Control MLD/6(Ki_S)
  Current Control/1(ModWave) -> ModWave/1
  Iab/1 -> Current Control/1(Iab)
  Kp_S/1 -> Speed Control MLD/5(Kp_S)
  Pos/1 -> Current Control/2(Pos)
  SpeedRef/1 -> RT6/1, RT3/1
  Mux/1 -> RT7/1
  RT2/1 -> Current Control/4(Idq_ref_PU)
  RT6/1 -> Current Control/5(SpeedRef)
  RT7/1 -> Current Control/3(Enable)
  RT1/1 -> Speed Control MLD/4(Speed_Meas_PU)
  RT3/1 -> Speed Control MLD/3(SpeedRef)
  Data Type Conversion/1 -> PWM_Enable/1
  RT5/1 -> Speed Control MLD/1(En_closedloop)
  RT4/1 -> Speed Control MLD/2(EnablePWM)
  Kp_i/1 -> Current Control/6(Kp_i)
  Ki_ixTcpu/1 -> Current Control/7(Ki_ixTcpu)

== system eVTOL_System/Motor Drive/Controller3/Controller_MIL/F28379D Firmware/Controller Algorithm/Speed and Pos Decoder ==
  QEP_Position_Count : Inport
  QEP_Index_Latch : Inport  Port=2
  Offset : Inport  Port=3
  Delay : Delay  DelayLength=1
  IIR Filter : mcbcontrolslib/IIR Filter  VariantControl=Low Pass Filter  VariantSelect=Low-pass  FilterConstantInputType=Specify via dialog  Filter_constant=0.01  advancedSettings=off  Ts=50e-6  cutOff_freq=32.1525
  IndexFinder : Subsystem
  Mechanical to Electrical Position : mcbpositiondecoderlib/Mechanical to Electrical Position  PolePairsInputType=Specify via dialog  NrPP=Maxon_645604_Np  selectedRange=Per unit  MechOfstInputType=Input port  mechOffsetIn=0  maxAngleIn=1  InputDataType=single  VariantSelect=floating-point
  NOT : Logic  Operator=NOT  AllPortsSameDT=off  OutDataTypeStr=boolean
  Quadrature Decoder : mcbpositiondecoderlib/Quadrature Decoder  EncoderSlitsPerRevolution=Maxon_Mile_Nslits  EncoderCountsPerSlit=4  CounterSize=16 bits  ExternalIndexCount=on  PositionUnit=Per unit  PositionDataType=single  ParameterInputType=off  CountsPerRevInverseDataType=single
  Speed Measurement : mcbpositiondecoderlib/Speed Measurement  PositionUnit=Per unit  PositionScalingDatatype=uint32  SpeedCalculationMode=Time interval for speed calculation  SampleTimeAsync=Ts_CPU  MaximumApplicationSpeed=6000  SpeedResolution=5e-6  DelayLength=20  MaximumMeasurableSpeed=29999  MeasurableSpeedResolution=1.397e-05  SpeedUnit=Per unit based on dialog  PerUnitSpeed=PU_System_N_base  SpeedDataType=single
  Theta_e : Outport  VectorParamsAs1DForOutWhenUnconnected=off
  speed : Outport  Port=2  VectorParamsAs1DForOutWhenUnconnected=off
  IndexFound : Outport  Port=3  InitialOutput=0  VectorParamsAs1DForOutWhenUnconnected=off
  wires:
  Mechanical to Electrical Position/1 -> Theta_e/1  "Pos"
  Speed Measurement/1 -> IIR Filter/1
  Quadrature Decoder/1 -> Speed Measurement/1, Mechanical to Electrical Position/1
  QEP_Position_Count/1 -> Quadrature Decoder/1
  Offset/1 -> Mechanical to Electrical Position/2
  IIR Filter/1 -> speed/1
  NOT/1 -> IndexFinder/Enable
  QEP_Index_Latch/1 -> IndexFinder/1(In1), Quadrature Decoder/2
  Delay/1 -> NOT/1
  IndexFinder/1(IndexFound) -> IndexFound/1, Delay/1

== system eVTOL_System/Battery System/BMS/HIL/Controller_100Cells/PLANT-Rx/Messages/Subsystem ==
  In1 : Inport
  In2 : Inport  Port=2
  3 : Inport  Port=3
  Bal_Cmd_Unpacking{,1..9} (10 alike) : slrealtimeutilitieslib/Bit Unpacking  SignExtend=on  MaskBitPatterns={[7:7] [6:6] [5:5] [4:4] [3:3] [2:2] [1:1] [0:0]}  MaskPackDataType=uint8  MaskPackDataSize=[1]  MaskUnpackDataTypes={'boolean', 'boolean', 'boolean', 'boolean', 'boolean', 'boolean', 'boolean', 'boolean'}  MaskUnpackDataSizes={[1] [1] [1] [1] [1] [1] [1] [1]}
  Demux : Demux
  Demux1 : Demux
  Demux2 : Demux  Outputs=2
  Demux3 : Demux  Outputs=2
  Mux : Mux  Inputs=76
  Terminator{,1..4} (5 alike) : Terminator
  Bal_Cmd_76Cells : Outport
  wires:
  In1/1 -> Demux/1
  Demux/1 -> Bal_Cmd_Unpacking/1
  Demux/2 -> Bal_Cmd_Unpacking1/1
  Demux/3 -> Bal_Cmd_Unpacking2/1
  Demux/4 -> Bal_Cmd_Unpacking3/1
  Demux1/1 -> Bal_Cmd_Unpacking4/1
  Demux1/2 -> Bal_Cmd_Unpacking5/1
  Demux1/3 -> Bal_Cmd_Unpacking6/1
  Demux1/4 -> Bal_Cmd_Unpacking7/1
  In2/1 -> Demux1/1
  3/1 -> Demux2/1
  Demux2/1 -> Demux3/1
  Demux3/1 -> Bal_Cmd_Unpacking8/1
  Demux3/2 -> Bal_Cmd_Unpacking9/1
  Bal_Cmd_Unpacking9/8 -> Terminator/1
  Bal_Cmd_Unpacking9/7 -> Terminator1/1
  Bal_Cmd_Unpacking9/6 -> Terminator2/1
  Bal_Cmd_Unpacking9/5 -> Terminator3/1
  Bal_Cmd_Unpacking/1 -> Mux/1
  Bal_Cmd_Unpacking/2 -> Mux/2
  Bal_Cmd_Unpacking/3 -> Mux/3
  Bal_Cmd_Unpacking/4 -> Mux/4
  Bal_Cmd_Unpacking/5 -> Mux/5
  Bal_Cmd_Unpacking/6 -> Mux/6
  Bal_Cmd_Unpacking/7 -> Mux/7
  Bal_Cmd_Unpacking/8 -> Mux/8
  Bal_Cmd_Unpacking1/1 -> Mux/9
  Bal_Cmd_Unpacking1/2 -> Mux/10
  Bal_Cmd_Unpacking1/3 -> Mux/11
  Bal_Cmd_Unpacking1/4 -> Mux/12
  Bal_Cmd_Unpacking1/5 -> Mux/13
  Bal_Cmd_Unpacking1/6 -> Mux/14
  Bal_Cmd_Unpacking1/7 -> Mux/15
  Bal_Cmd_Unpacking1/8 -> Mux/16
  Bal_Cmd_Unpacking2/1 -> Mux/17
  Bal_Cmd_Unpacking2/2 -> Mux/18
  Bal_Cmd_Unpacking2/3 -> Mux/19
  Bal_Cmd_Unpacking2/4 -> Mux/20
  Bal_Cmd_Unpacking2/5 -> Mux/21
  Bal_Cmd_Unpacking2/6 -> Mux/22
  Bal_Cmd_Unpacking2/7 -> Mux/23
  Bal_Cmd_Unpacking2/8 -> Mux/24
  Bal_Cmd_Unpacking3/1 -> Mux/25
  Bal_Cmd_Unpacking3/2 -> Mux/26
  Bal_Cmd_Unpacking3/3 -> Mux/27
  Bal_Cmd_Unpacking3/4 -> Mux/28
  Bal_Cmd_Unpacking3/5 -> Mux/29
  Bal_Cmd_Unpacking3/6 -> Mux/30
  Bal_Cmd_Unpacking3/7 -> Mux/31
  Bal_Cmd_Unpacking3/8 -> Mux/32
  Bal_Cmd_Unpacking4/1 -> Mux/33
  Bal_Cmd_Unpacking4/2 -> Mux/34
  Bal_Cmd_Unpacking4/3 -> Mux/35
  Bal_Cmd_Unpacking4/4 -> Mux/36
  Bal_Cmd_Unpacking4/5 -> Mux/37
  Bal_Cmd_Unpacking4/6 -> Mux/38
  Bal_Cmd_Unpacking4/7 -> Mux/39
  Bal_Cmd_Unpacking4/8 -> Mux/40
  Bal_Cmd_Unpacking5/1 -> Mux/41
  Bal_Cmd_Unpacking5/2 -> Mux/42
  Bal_Cmd_Unpacking5/3 -> Mux/43
  Bal_Cmd_Unpacking5/4 -> Mux/44
  Bal_Cmd_Unpacking5/5 -> Mux/45
  Bal_Cmd_Unpacking5/6 -> Mux/46
  Bal_Cmd_Unpacking5/7 -> Mux/47
  Bal_Cmd_Unpacking5/8 -> Mux/48
  Bal_Cmd_Unpacking6/1 -> Mux/49
  Bal_Cmd_Unpacking6/2 -> Mux/50
  Bal_Cmd_Unpacking6/3 -> Mux/51
  Bal_Cmd_Unpacking6/4 -> Mux/52
  Bal_Cmd_Unpacking6/5 -> Mux/53
  Bal_Cmd_Unpacking6/6 -> Mux/54
  Bal_Cmd_Unpacking6/7 -> Mux/55
  Bal_Cmd_Unpacking6/8 -> Mux/56
  Bal_Cmd_Unpacking7/1 -> Mux/57
  Bal_Cmd_Unpacking7/2 -> Mux/58
  Bal_Cmd_Unpacking7/3 -> Mux/59
  Bal_Cmd_Unpacking7/4 -> Mux/60
  Bal_Cmd_Unpacking7/5 -> Mux/61
  Bal_Cmd_Unpacking7/6 -> Mux/62
  Bal_Cmd_Unpacking7/7 -> Mux/63
  Bal_Cmd_Unpacking7/8 -> Mux/64
  Bal_Cmd_Unpacking8/5 -> Mux/69
  Bal_Cmd_Unpacking8/4 -> Mux/68
  Bal_Cmd_Unpacking8/6 -> Mux/70
  Bal_Cmd_Unpacking8/3 -> Mux/67
  Bal_Cmd_Unpacking8/7 -> Mux/71
  Bal_Cmd_Unpacking8/2 -> Mux/66
  Bal_Cmd_Unpacking8/8 -> Mux/72
  Bal_Cmd_Unpacking8/1 -> Mux/65
  Bal_Cmd_Unpacking9/4 -> Mux/76
  Bal_Cmd_Unpacking9/3 -> Mux/75
  Bal_Cmd_Unpacking9/2 -> Mux/74
  Bal_Cmd_Unpacking9/1 -> Mux/73
  Mux/1 -> Bal_Cmd_76Cells/1
  Demux2/2 -> Terminator4/1
